simulink model "basic_consensus_average"  (R2017a)
settings: Solver=VariableStepAuto  StartTime=0.0  StopTime=1000  RelTol=1e-3
values from neighbouring files (symbols this model uses):
  A = double((A + A') /2 > 0)    [init.m]    (also in init_consensus.m = ones(n) - eye(n); init_trust_consensus.m = ones(n) - eye(n))
  comm_type = 2    [init_consensus.m]    (also in init_trust_consensus.m)
  event_based = 1    [init_consensus.m]    (also in init_consensus_15.m = 0; init_trust_consensus.m; matlab.mat; test100.m = 0)
  n = input(prompt)    [init.m]    (also in init_consensus.m = 4; init_consensus_15.m = 15; init_mussels.m = 5; init_mussels_2.m = 5)
  sigma0 = zeros(n,n)    [init_trust_consensus.m]
  Td = 2    [init_consensus.m]    (also in init_trust_consensus.m = 5)
  x0 = [0 30 50 100]    [init_consensus.m]    (also in init_consensus_15.m = [19    14   135   199   238    33   145   120     3    86   ; init_trust_consensus.m; matlab.mat = [50 100 30 150 0]; test100.m = 255.*rand(n,1))
  zeta0 = zeros(n, n)    [init_trust_consensus.m]
undefined symbols (not defined in the file or in its folder): DiscIntNeverNeededParam
settings Model: Creator=Barbara  LastModifiedBy=Annie

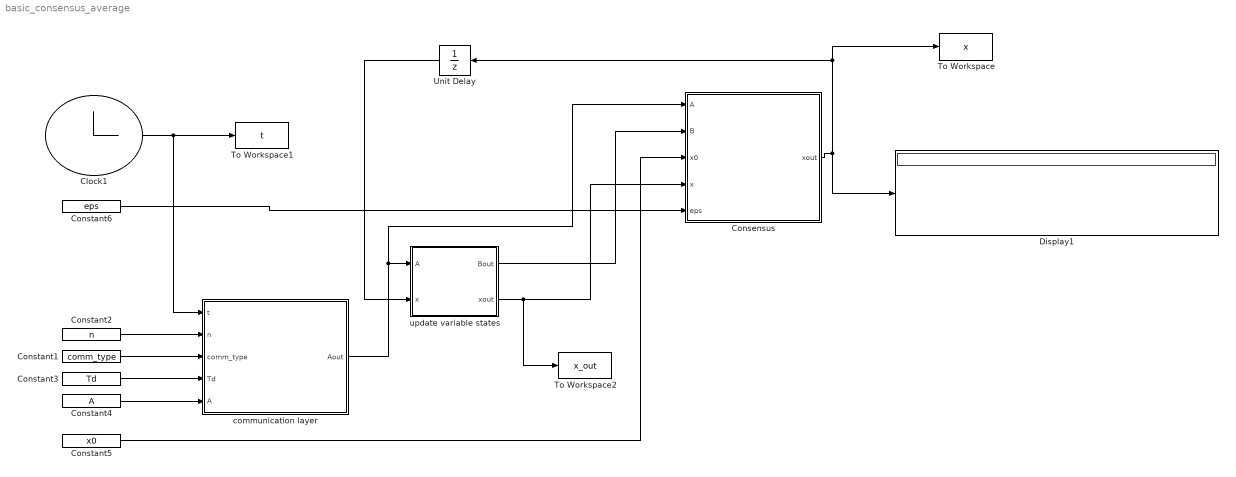
== system basic_consensus_average ==
  Clock1 : Clock
  Consensus : Subsystem
  Constant1 : Constant  Value=comm_type  OutMin=[1]  OutMax=[2]
  Constant2 : Constant  Value=n  OutMin=[1]  OutMax=200
  Constant3 : Constant  Value=Td  OutMin=[1]
  Constant4 : Constant  Value=A  OutMin=[0]  OutMax=[1]
  Constant5 : Constant  Value=x0
  Constant6 : Constant  Value=eps  OutMin=[0]  OutMax=[1]
  Display1 : Display
  To Workspace : ToWorkspace  VariableName=x  SampleTime=-1
  To Workspace1 : ToWorkspace  VariableName=t  SampleTime=-1
  To Workspace2 : ToWorkspace  VariableName=x_out  SampleTime=-1
  Unit Delay : UnitDelay  InitialCondition=-1  SampleTime=-1
  communication layer : Subsystem
  update variable states : Subsystem
  wires:
  Clock1/1 -> To Workspace1/1, communication layer/1(t)
  Constant1/1 -> communication layer/3(comm_type)
  Constant2/1 -> communication layer/2(n)
  Constant3/1 -> communication layer/4(Td)
  Constant4/1 -> communication layer/5(A)
  Constant5/1 -> Consensus/3(x0)
  Consensus/1(xout) -> Display1/1, To Workspace/1, Unit Delay/1
  Constant6/1 -> Consensus/5(eps)
  communication layer/1(Aout) -> Consensus/1(A), update variable states/1(A)
  update variable states/2(xout) -> To Workspace2/1, Consensus/4(x)
  update variable states/1(Bout) -> Consensus/2(B)
  Unit Delay/1 -> update variable states/2(x)

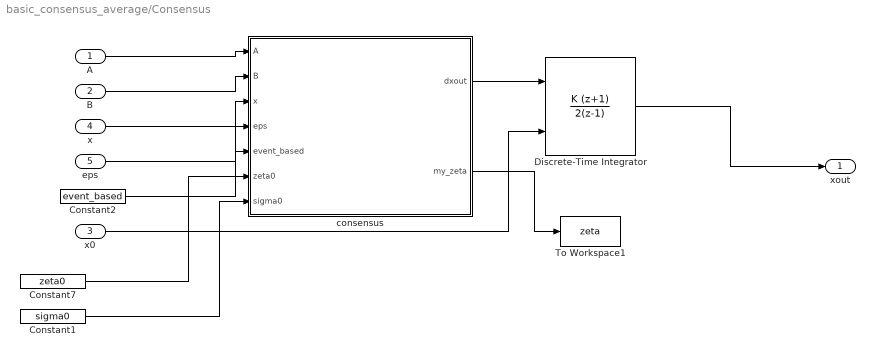
== system basic_consensus_average/Consensus ==
  A : Inport
  B : Inport  Port=2
  x0 : Inport  Port=3
  x : Inport  Port=4
  eps : Inport  Port=5
  Constant1 : Constant  Value=sigma0  OutMin=[0]  OutMax=1
  Constant2 : Constant  Value=event_based  OutMin=[0]  OutMax=[1]
  Constant7 : Constant  Value=zeta0  OutMin=[0]  OutMax=1
  Discrete-Time Integrator : DiscreteIntegrator  IntegratorMethod=Accumulation: Trapezoidal  InitialConditionSource=external  InitialConditionSetting=State (most efficient)  ICPrevOutput=DiscIntNeverNeededParam  ICPrevScaledInput=DiscIntNeverNeededParam
  To Workspace1 : ToWorkspace  VariableName=zeta  SampleTime=-1
  consensus : MATLAB Function  TreatAsAtomicUnit=on
  xout : Outport
  wires:
  x0/1 -> Discrete-Time Integrator/2
  consensus/1(dxout) -> Discrete-Time Integrator/1
  eps/1 -> consensus/4(eps)
  B/1 -> consensus/2(B)
  x/1 -> consensus/3(x)
  A/1 -> consensus/1(A)
  Constant2/1 -> consensus/5(event_based)
  Discrete-Time Integrator/1 -> xout/1
  Constant7/1 -> consensus/6(zeta0)
  Constant1/1 -> consensus/7(sigma0)
  consensus/2(my_zeta) -> To Workspace1/1

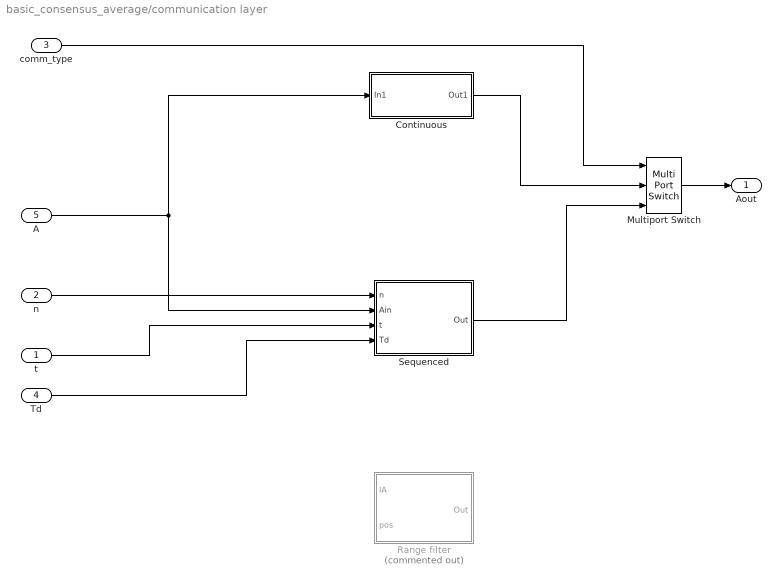
== system basic_consensus_average/communication layer ==
  t : Inport
  n : Inport  Port=2
  comm_type : Inport  Port=3
  Td : Inport  Port=4
  A : Inport  Port=5
  Continuous : Subsystem
  Multiport Switch : MultiPortSwitch  Inputs=2  DiagnosticForDefault=Warning  OutDataTypeStr=Inherit: Inherit via back propagation
  Range filter : Subsystem  Commented=on
  Sequenced : Subsystem
  Aout : Outport
  wires:
  A/1 -> Sequenced/2(Ain), Continuous/1(In1)
  t/1 -> Sequenced/3(t)
  Multiport Switch/1 -> Aout/1
  Sequenced/1(Out) -> Multiport Switch/3
  n/1 -> Sequenced/1(n)
  Continuous/1(Out1) -> Multiport Switch/2
  comm_type/1 -> Multiport Switch/1
  Td/1 -> Sequenced/4(Td)

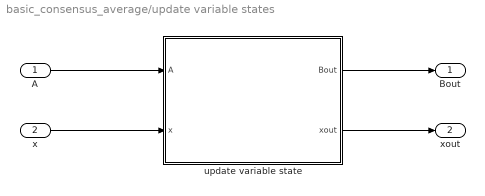
== system basic_consensus_average/update variable states ==
  A : Inport
  x : Inport  Port=2
  update variable state : MATLAB Function  TreatAsAtomicUnit=on
  Bout : Outport
  xout : Outport  Port=2
  wires:
  A/1 -> update variable state/1(A)
  x/1 -> update variable state/2(x)
  update variable state/1(Bout) -> Bout/1
  update variable state/2(xout) -> xout/1

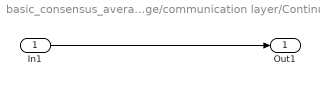
== system basic_consensus_average/communication layer/Continuous ==
  In1 : Inport
  Out1 : Outport
  wires:
  In1/1 -> Out1/1

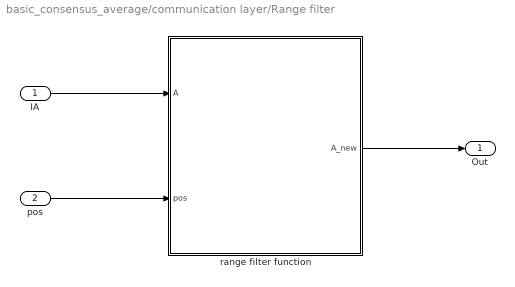
== system basic_consensus_average/communication layer/Range filter ==
  IA : Inport
  pos : Inport  Port=2
  range filter function : MATLAB Function  TreatAsAtomicUnit=on
  Out : Outport
  wires:
  IA/1 -> range filter function/1(A)
  pos/1 -> range filter function/2(pos)
  range filter function/1(A_new) -> Out/1

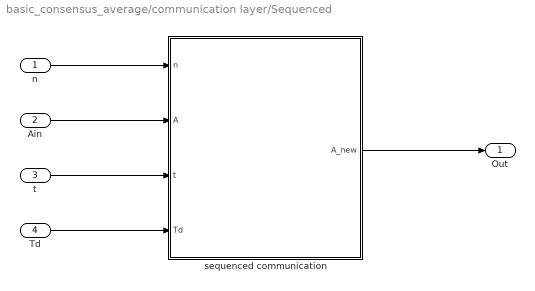
== system basic_consensus_average/communication layer/Sequenced ==
  n : Inport
  Ain : Inport  Port=2
  t : Inport  Port=3
  Td : Inport  Port=4
  sequenced communication : MATLAB Function  TreatAsAtomicUnit=on
  Out : Outport
  wires:
  n/1 -> sequenced communication/1(n)
  Ain/1 -> sequenced communication/2(A)
  sequenced communication/1(A_new) -> Out/1
  t/1 -> sequenced communication/3(t)
  Td/1 -> sequenced communication/4(Td)

== matlab function basic_consensus_average/communication layer/Sequenced/sequenced communication ==
  data: n input; A input; t input; Td input; A_new output
function A_new = sequenced_comms_filter_A(n,A,t,Td)
    persistent lastComm;
    c = floor(mod(t,(n*Td))/Td) + 1;
    calc = true;
    comm  = zeros(1,n);
    
    if isempty(lastComm)
        lastComm = c;
        calc = true;
    else
        if lastComm == c
            calc = false;
        else
            lastComm = c;
            calc = true;
        end
    end
    
    if calc
        comm(floor(mod(t,(n*Td))/Td) + 1) = 1;
        mask = repmat(comm,size(A,1),1);
        A_new = A .* mask;
    else
        A_new = zeros(size(A));
    end
  end

== matlab function basic_consensus_average/communication layer/Range filter/range filter function ==
  data: A input; pos input; A_new output
function A_new = range_filter_A(A,pos)
    A_new = A;
  end

== matlab function basic_consensus_average/Consensus/consensus ==
  data: A input; B input; x input; dxout output; eps input; event_based input; zeta0 input; sigma0 input; my_zeta output
function [dxout, my_zeta] = consensus(A, B, x, eps, event_based, zeta0, sigma0)
    
    % initializing trust matrix zeta
    persistent zeta;
    
    % if zeta is empty, initial value of
    % zeta is zeta0 (defined in init)
    if isempty(zeta)
        zeta = zeta0;
    end
    
    % because persistent variable
    % can't be output of a function
    my_zeta = zeros(size(zeta));
    dxout=zeros(size(B,1),1);
    calc=1;
    if event_based
        if isempty(find(A,1))
            calc=0;
        end
    end
    
    if calc
        % svaki i
        for i=1:size(x,1)
            % updejta povjerenje prema j
            for j=1:size(x,1)
                if i~=j
                    % if agents are excahnging floats, remove the round()
                    dxout(i) = dxout(i) + eps * B(i,j)*(round(x(i,j)) - x(i,i));
                    
                    % calculating measuring error
                    delta = round(x(i,j)) - x(i,i);
                    
                    % observation function (part of the trust based solely
                    % on their observation of their neighbour)
                    observ_func = exp(delta^2/sigma0(i,j)^2);
                    
                    % change of zeta 
                    dzeta = sign(observ_func - zeta(i,j));
                    
                    % adding that change to defined zeta
                    zeta(i,j) = zeta(i,j) + dzeta;
                end
            end
        end
    end
my_zeta = zeta;

== matlab function basic_consensus_average/update variable states/update variable state ==
  data: A input; Bout output; x input; xout output
function [Bout,xout] = update_var_states(A,x)
    persistent xcomm;
    if isempty(xcomm)
        xcomm = zeros(size(A));
    end
    
    persistent B;
    if isempty(B)
        B = zeros(size(A));
    end    
    if length(find(~all(B==0))) == size(x,1)
        %reset
        B = zeros(size(A));
    end
    
    % because fo the delay of the signal
    if max(x)==-1
        xout = zeros(size(A));
        Bout = zeros(size(A));
        return;
    end
    B = double((B + A)~=0);
    Bout=B;
    
    % find out who is sending a message atm
    mask = all(A==0);
    index = find(~mask);
    if ~isempty(index)
        for j = 1: length(index)
            i = index(j);
            % update communicated values
            xcomm(:,i) = repmat(x(i),1,size(xcomm,1));
            xcomm(i,i) = 0;
        end
    end
    
    if length(find(~all(B==0))) ~= size(x,1)
        xout = zeros(size(A));
        return;
    end
    xout = xcomm + diag(x)
